simulink model "WCRC_mu_test"  (R2023b)
settings: Solver=FixedStepAuto  StartTime=0.0  StopTime=50  FixedStep=0.001  RelTol=1e-3
libraries: Solver_SF x1
settings Model: Creator=황수빈  LastModifiedBy=황수빈

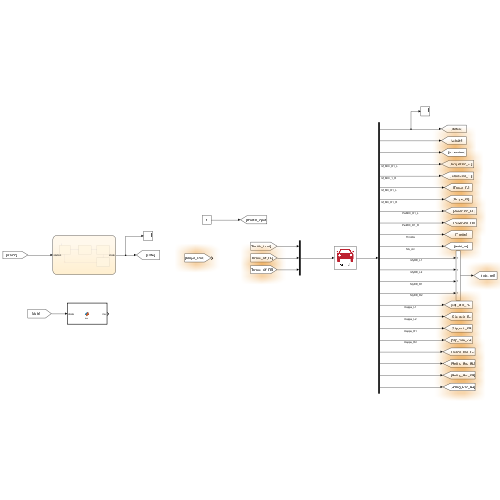
[thumbnail: Simulink's stored preview of the top-level diagram]
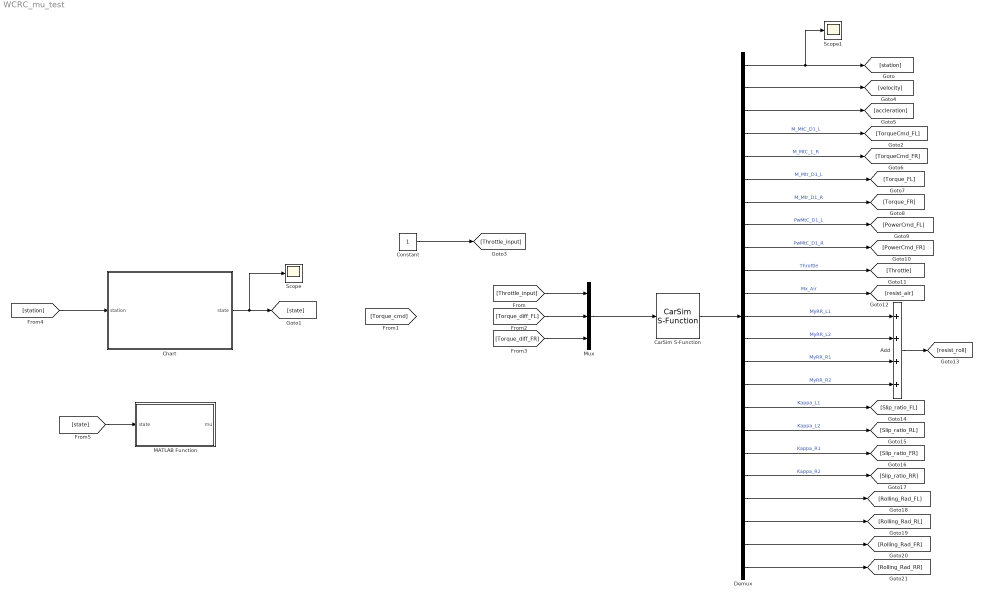
== system WCRC_mu_test ==
  Add : Sum  Inputs=++++
  CarSim S-Function : Solver_SF/CarSim S-Function  Priority=1  SIMFILE=simfile.sim  Run_RTs=off  vs_state_ind=Run  StopMode_ind=Vehicle Model
  Chart : Stateflow chart  TreatAsAtomicUnit=on
  Constant : Constant
  Demux : Demux  Outputs=23
  MATLAB Function : MATLAB Function  TreatAsAtomicUnit=on
  Mux : Mux  Inputs=3
  Scope : Scope
  Scope1 : Scope
  wires:
  CarSim S-Function/1 -> Demux/1
  Demux/1 -> Scope1/1, [station]
  Mux/1 -> CarSim S-Function/1
  [Throttle_input] -> Mux/1
  Constant/1 -> [Throttle_input]
  [Torque_diff_FL] -> Mux/2
  [Torque_diff_FR] -> Mux/3
  Demux/2 -> [velocity]
  Demux/3 -> [accleration]
  Demux/4 -> [TorqueCmd_FL]  "M_MtC_D1_L"
  Demux/5 -> [TorqueCmd_FR]  "M_MtC_1_R"
  Demux/6 -> [Torque_FL]  "M_Mtr_D1_L"
  Demux/7 -> [Torque_FR]  "M_Mtr_D1_R"
  Demux/8 -> [PowerCmd_FL]  "PwMtC_D1_L"
  Demux/9 -> [PowerCmd_FR]  "PwMtC_D1_R"
  Demux/10 -> [Throttle]  "Throttle"
  Demux/11 -> [resist_air]  "Mx_Air"
  Demux/12 -> Add/1  "MyRR_L1"
  Demux/13 -> Add/2  "MyRR_L2"
  Demux/14 -> Add/3  "MyRR_R1"
  Demux/15 -> Add/4  "MyRR_R2"
  Add/1 -> [resist_roll]
  Demux/16 -> [Slip_ratio_FL]  "Kappa_L1"
  Demux/17 -> [Slip_ratio_RL]  "Kappa_L2"
  Demux/18 -> [Slip_ratio_FR]  "Kappa_R1"
  Demux/19 -> [Slip_ratio_RR]  "Kappa_R2"
  [station] -> Chart/1(station)
  Chart/1(state) -> Scope/1, [state]
  [state] -> MATLAB Function/1(state)
  Demux/20 -> [Rolling_Rad_FL]
  Demux/21 -> [Rolling_Rad_RL]
  Demux/22 -> [Rolling_Rad_FR]
  Demux/23 -> [Rolling_Rad_RR]

== matlab function WCRC_mu_test/MATLAB Function ==
  data: state input; mu output
function mu = fcn(state)

mu = state;

== stateflow chart WCRC_mu_test/Chart ==
  state INIT
    en:
    state=0;
  state Ice
    en:
    state=1;
  state Concrete
    en:
    state=2;
  state SplitMu
    en:
    state=3;
  (default) -> INIT
  INIT -> Ice : [station==100]
  Ice -> Concrete : [station==405]
  (junction 17) -> INIT
  Concrete -> SplitMu : [station==738]
  SplitMu -> (junction 17) : [station==1040]
  data: station input; state output
